simulink model "PI"  (R2022b)
settings: Solver=VariableStepAuto  StartTime=0.0  StopTime=10.0  RelTol=1e-3
settings Model: Creator=Vikhyath  LastModifiedBy=Vikhyath

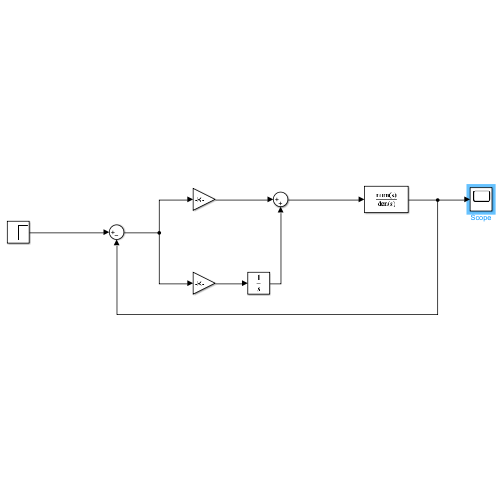
[thumbnail: Simulink's stored preview of the top-level diagram]
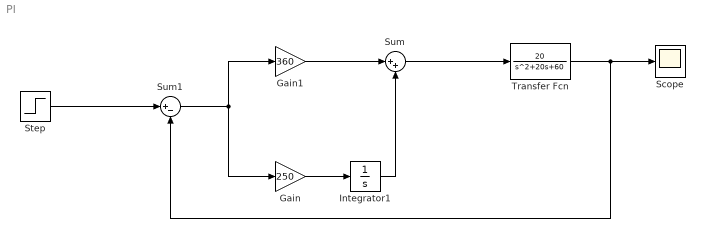
== system PI ==
  Gain : Gain  Gain=250
  Gain1 : Gain  Gain=360
  Integrator1 : Integrator
  Scope : Scope
  Step : Step  Time=0  SampleTime=0
  Sum : Sum  Inputs=|++
  Sum1 : Sum  Inputs=|+-
  Transfer Fcn : TransferFcn  Numerator=[20]  Denominator=[1 20 60]
  wires:
  Step/1 -> Sum1/1
  Gain/1 -> Integrator1/1
  Sum1/1 -> Gain/1, Gain1/1
  Gain1/1 -> Sum/1
  Integrator1/1 -> Sum/2
  Sum/1 -> Transfer Fcn/1
  Transfer Fcn/1 -> Sum1/2, Scope/1
